simulink model "CSI_0313_SDC"  (R2019b)
settings: Solver=FixedStepDiscrete  StartTime=0.0  StopTime=Tstop  FixedStep=Tdelt  MaxStep=1e-4  RelTol=1e-3
values from neighbouring files (symbols this model uses):
  C = 12e-6    (= 1.2e-05)    [Inputparameter.m]
  Cdc = 4.76*10^-3    (= 0.00476)    [Inputparameter.m]
  Cemc = 1.5e-6    (= 1.5e-06)    [Inputparameter.m]
  enb = 0    [Run.m]
  fanalog = 7000    [Run.m]
  fTs = Update/18000    (= 0.000111111111111)    [Run.m]
  Ibase = 43*sqrt(2)    [Inputparameter.m]
  K120 = 0.0    (= 0)    [Run.m]
  K21 = 0.0    (= 0)    [Run.m]
  K5 = 0.0    (= 0)    [Run.m]
  K7 = 0.0    (= 0)    [Run.m]
  Kipll = 1.0    (= 1)    [Run.m]
  Klim = 1.03    [Run.m]
  Kpll = 20.0    (= 20)    [Run.m]
  Kpr = 0.9*Ibase/(Vbase)    [Run.m]
  Lgrid = 7.717e-4*10    (= 0.007717)    [Run.m]
  Lline = 60e-6    (= 6e-05)    [Inputparameter.m]
  Lpwm = 184.8e-6    (= 0.0001848)    [Inputparameter.m]
  mode = 1    [Run.m]
  Nsw = 18000/fbase    [Run.m]
  Qbpf = 1.0    (= 1)    [Run.m]
  Qpr = 1.0    (= 1)    [Run.m]
  Qs = 1    [Run.m]
  Rc = 10e-3    (= 0.01)    [Inputparameter.m]
  Remc = 1e-3    (= 0.001)    [Inputparameter.m]
  Rgrid = 2*pi*fbase*Lgrid/XR    [Run.m]
  Rline = 4.95e-3    (= 0.00495)    [Inputparameter.m]
  Rpre = 2.2    [Inputparameter.m]
  Rpwm = 6.2e-3    (= 0.0062)    [Inputparameter.m]
  Tdelt = (fTs)/(200*Update)    (= 2.77777777778e-07)    [Run.m]
  Tdt = 1.27e-6    (= 1.27e-06)    [Run.m]
  tstart = 0.2    [Run.m]
  Update = 2    [Run.m]
  Vbase = 400*sqrt(2/3)    [Inputparameter.m]
undefined symbols (not defined in the file or in its folder): sigbuilder_block
libraries: powerlib x54
(part 3 of 4)

== matlab function CSI_0313_SDC/AIP1/Subsystem7/Pos&Neg seq extract in subsystem /IIR_BPF_Re1 ==
  data: u input; fn input; fQ parameter; y output; fTs parameter; iMode parameter
function y =IIR_2rd(u, fn, fQ, fTs, iMode)
    % Second order transfer function used for LPF and BPF
    % y[n] = (fa1*x[n]+fa2*x[n-1]+fa3*x[n-2]-fb2*y[n-1]-fb3*y[n-2])/fb1
    % u:  error input
    % fn:  Natural frequency
    % fQ:   Quality factor
    % fTs:  Sampling time
    % iMode: Mode Selection
    % iMode=1 used as generalized 2nd-order LPF, LPF(s)=wn^2/(s^2+wn/Q*s+wn^2)
    % iMode=2 used as 2nd-order LPF in SOGI, SOGI_LPF(s)=(wn^2/Q)/(s^2+wn/Q*s+wn^2)
    % iMode=3 used as 2nd-order BPF in SOGI, SOGI_BPF(s)=(wn*s/Q)/(s^2+wn/Q*s+wn^2)
    
    persistent t;
    
    if isempty(t)
        t = zeros(2,3);
    end
    
    wn = 2*pi*fn;
    wc = wn/fQ;

    fT1 = wc*wn*fTs*fTs; 
    fT2 = 2*wc*fTs;
    fT3 = (wn*fTs)^2;
    
    fb1 = fT3+fT2+4;
    fb2 = 2*fT3-8;
    fb3 = fT3-fT2+4;
    
    if (iMode ==1)
        fa1 = fT3;
        fa2 = 2*fT3;
        fa3 = fT3;
    elseif (iMode ==2)
        fa1 = fT1;
        fa2 = 2*fT1;
        fa3 = fT1;
    else
        fa1 = fT2;
        fa2 = 0;
        fa3 = -fT2;
    end
%     if(Trigs > 0)
        t(1,1) = u;        
        t(2,1) = (fa1*t(1,1)+fa2*t(1,2)+fa3*t(1,3)-fb2*t(2,2)-fb3*t(2,3))/fb1;
    
        t(1,3) = t(1,2);
        t(1,2) = t(1,1);
        
        t(2,3) = t(2,2);
        t(2,2) = t(2,1);
%     else
%         t(1,1) = t(1,1);        
%         t(2,1) = t(2,1);
%     
%         t(1,3) = t(1,3);
%         t(1,2) = t(1,2);
%         
%         t(2,3) = t(2,3);
%         t(2,2) = t(2,2);
%     end
    
    y = t(2,1);    
end

== matlab function CSI_0313_SDC/AIP1/Subsystem7/Pos&Neg seq extract in subsystem /IIR_LPF_Im ==
  data: u input; fn input; fQ parameter; y output; fTs parameter; iMode parameter
function y =IIR_2rd(u, fn, fQ, fTs, iMode)
    % Second order transfer function used for LPF and BPF
    % y[n] = (fa1*x[n]+fa2*x[n-1]+fa3*x[n-2]-fb2*y[n-1]-fb3*y[n-2])/fb1
    % u:  error input
    % fn:  Natural frequency
    % fQ:   Quality factor
    % fTs:  Sampling time
    % iMode: Mode Selection
    % iMode=1 used as generalized 2nd-order LPF, LPF(s)=wn^2/(s^2+wn/Q*s+wn^2)
    % iMode=2 used as 2nd-order LPF in SOGI, SOGI_LPF(s)=(wn^2/Q)/(s^2+wn/Q*s+wn^2)
    % iMode=3 used as 2nd-order BPF in SOGI, SOGI_BPF(s)=(wn*s/Q)/(s^2+wn/Q*s+wn^2)
    
    persistent t;
    
    if isempty(t)
        t = zeros(2,3);
    end
    
    wn = 2*pi*fn;
    wc = wn/fQ;

    fT1 = wc*wn*fTs*fTs; 
    fT2 = 2*wc*fTs;
    fT3 = (wn*fTs)^2;
    
    fb1 = fT3+fT2+4;
    fb2 = 2*fT3-8;
    fb3 = fT3-fT2+4;
    
    if (iMode ==1)
        fa1 = fT3;
        fa2 = 2*fT3;
        fa3 = fT3;
    elseif (iMode ==2)
        fa1 = fT1;
        fa2 = 2*fT1;
        fa3 = fT1;
    else
        fa1 = fT2;
        fa2 = 0;
        fa3 = -fT2;
    end
        
%    if(Trigs > 0)
        t(1,1) = u;        
        t(2,1) = (fa1*t(1,1)+fa2*t(1,2)+fa3*t(1,3)-fb2*t(2,2)-fb3*t(2,3))/fb1;
    
        t(1,3) = t(1,2);
        t(1,2) = t(1,1);
        
        t(2,3) = t(2,2);
        t(2,2) = t(2,1);
%     else
%         t(1,1) = t(1,1);        
%         t(2,1) = t(2,1);
%     
%         t(1,3) = t(1,3);
%         t(1,2) = t(1,2);
%         
%         t(2,3) = t(2,3);
%         t(2,2) = t(2,2);
%     end
%     
    y = t(2,1);    
end

== matlab function CSI_0313_SDC/AIP1/Subsystem7/Current Limitation pu Standard/PI Ctrl ==
  data: err input; y output; fKI parameter; fMinLmt parameter; fTs parameter; fMaxLmt parameter; fKP parameter
function y = PICtrl(err, fKI, fMinLmt, fTs, fMaxLmt, fKP)
    % y[n] = y[n-1] + KP*(x[n]-x[n-1]) + (KP*KI*TS*0.5)*(x[n]+x[n-1])
    % err:  error input
    % fKP:   Proportional gain
    % fKI:   Integral Coefficient
    % fMinLmt: Minimum limitation
    % fMaxLmt: Maximum limitation
    % fTs:  Sampling time
    
    % t(1,2) stores x[n],x[n-1]; t(2,2) stores y[n],y[n-1]
    persistent t;      
    if isempty(t)           % Initialization
        t = zeros(2,2);
    end
    
%     if(Trig > 0)
        t(1,1) = err;
        t(2,1) = t(2,2) + fKP*(t(1,1)-t(1,2)) + fKP*fKI*0.5*(t(1,1)+t(1,2))*fTs;   
    
        if (t(2,1) < fMinLmt)
            t(2,1) = fMinLmt;
        elseif (t(2,1) > fMaxLmt)
            t(2,1) = fMaxLmt;
        end
    
        t(1,2) = t(1,1);
        t(2,2) = t(2,1);
%     else
%         t(1,1) = t(1,1);
%         t(2,1) = t(2,1);      
%         t(1,2) = t(1,2);
%         t(2,2) = t(2,2);
%     end
    y = t(2,1);
end

== matlab function CSI_0313_SDC/Programmal Grid/Programmal Grid  ==
  data: ua output; ub output; uc output; Tdelt parameter; K5 parameter; K7 parameter; K21 parameter; K120 parameter; t input
function [ua, ub, uc] = fcn(Tdelt,K5, K7, K21,K120,t)
persistent theta; 
 % Initialization
 if isempty(theta)           
    theta = pi/2;
 end 

f = 50;
Vm = 400*sqrt(2/3);
Tflt = 0.2;             %% fault duration time[s]
Vsag = 0.05 * Vm;        %% voltage level configuration during the fault
theta = theta + 2*pi*f*Tdelt;
if(theta >= 2*pi)
    theta = theta-2*pi;
end

Tinrpt = 12.21;
if (t < Tinrpt)
    Vol = Vm;
elseif (t>=Tinrpt && t<(Tinrpt+0.004))  %% the fault starts and ends in 4ms
    Vol = Vm-(t-Tinrpt)*(Vm - Vsag)/0.004;
elseif (t>=Tinrpt && t<(Tinrpt+0.004+Tflt)) %% the fault sustain Tflt[s]
    Vol = Vsag;
elseif (t>=(Tinrpt+0.004+Tflt) && t< (Tinrpt+0.008+Tflt))  %% the fault recoverys in 4ms
    Vol = Vsag+(t-(Tinrpt+0.004+Tflt))*(Vm - Vsag)/0.004;
else
    Vol = Vm;
end

ua = Vol*sin(theta)+K5*Vm*sin(5.0*theta)+K7*Vm*sin(7.0*theta)+K21*Vm*sin(21.0*theta)+K120*Vm*sin(120.0*theta);
ub = Vol*sin(theta-2*pi/3)+K5*Vm*sin(5.0*(theta-2*pi/3))+K7*Vm*sin(7.0*(theta-2*pi/3))+K120*Vm*sin(120.0*(theta-2*pi/3));
uc = Vol*sin(theta+2*pi/3)+K5*Vm*sin(5.0*(theta+2*pi/3))+K7*Vm*sin(7.0*(theta+2*pi/3))+K120*Vm*sin(120.0*(theta+2*pi/3));

end

== matlab function CSI_0313_SDC/AIP1/Subsystem7/Pos&Neg seq extract in subsystem /IIR_LPF_Re1 ==
  data: u input; fn input; fQ parameter; y output; fTs parameter; iMode parameter
function y =IIR_2rd(u, fn, fQ, fTs, iMode)
    % Second order transfer function used for LPF and BPF
    % y[n] = (fa1*x[n]+fa2*x[n-1]+fa3*x[n-2]-fb2*y[n-1]-fb3*y[n-2])/fb1
    % u:  error input
    % fn:  Natural frequency
    % fQ:   Quality factor
    % fTs:  Sampling time
    % iMode: Mode Selection
    % iMode=1 used as generalized 2nd-order LPF, LPF(s)=wn^2/(s^2+wn/Q*s+wn^2)
    % iMode=2 used as 2nd-order LPF in SOGI, SOGI_LPF(s)=(wn^2/Q)/(s^2+wn/Q*s+wn^2)
    % iMode=3 used as 2nd-order BPF in SOGI, SOGI_BPF(s)=(wn*s/Q)/(s^2+wn/Q*s+wn^2)
    
    persistent t;
    
    if isempty(t)
        t = zeros(2,3);
    end
    
    wn = 2*pi*fn;
    wc = wn/fQ;

    fT1 = wc*wn*fTs*fTs; 
    fT2 = 2*wc*fTs;
    fT3 = (wn*fTs)^2;
    
    fb1 = fT3+fT2+4;
    fb2 = 2*fT3-8;
    fb3 = fT3-fT2+4;
    
    if (iMode ==1)
        fa1 = fT3;
        fa2 = 2*fT3;
        fa3 = fT3;
    elseif (iMode ==2)
        fa1 = fT1;
        fa2 = 2*fT1;
        fa3 = fT1;
    else
        fa1 = fT2;
        fa2 = 0;
        fa3 = -fT2;
    end
        
%    if(Trigs > 0)
        t(1,1) = u;        
        t(2,1) = (fa1*t(1,1)+fa2*t(1,2)+fa3*t(1,3)-fb2*t(2,2)-fb3*t(2,3))/fb1;
    
        t(1,3) = t(1,2);
        t(1,2) = t(1,1);
        
        t(2,3) = t(2,2);
        t(2,2) = t(2,1);
%     else
%         t(1,1) = t(1,1);        
%         t(2,1) = t(2,1);
%     
%         t(1,3) = t(1,3);
%         t(1,2) = t(1,2);
%         
%         t(2,3) = t(2,3);
%         t(2,2) = t(2,2);
%     end
    
    y = t(2,1);    
end

== matlab function CSI_0313_SDC/AIP1/Subsystem7/Pos&Neg seq extract in subsystem 1/IIR_BPF_Im ==
  data: u input; fn input; fQ parameter; y output; fTs parameter; iMode parameter
function y =IIR_2rd(u, fn, fQ, fTs, iMode)
    % Second order transfer function used for LPF and BPF
    % y[n] = (fa1*x[n]+fa2*x[n-1]+fa3*x[n-2]-fb2*y[n-1]-fb3*y[n-2])/fb1
    % u:  error input
    % fn:  Natural frequency
    % fQ:   Quality factor
    % fTs:  Sampling time
    % iMode: Mode Selection
    % iMode=1 used as generalized 2nd-order LPF, LPF(s)=wn^2/(s^2+wn/Q*s+wn^2)
    % iMode=2 used as 2nd-order LPF in SOGI, SOGI_LPF(s)=(wn^2/Q)/(s^2+wn/Q*s+wn^2)
    % iMode=3 used as 2nd-order BPF in SOGI, SOGI_BPF(s)=(wn*s/Q)/(s^2+wn/Q*s+wn^2)
    
    persistent t;
    
    if isempty(t)
        t = zeros(2,3);
    end
    
    wn = 2*pi*fn;
    wc = wn/fQ;

    fT1 = wc*wn*fTs*fTs; 
    fT2 = 2*wc*fTs;
    fT3 = (wn*fTs)^2;
    
    fb1 = fT3+fT2+4;
    fb2 = 2*fT3-8;
    fb3 = fT3-fT2+4;
    
    if (iMode ==1)
        fa1 = fT3;
        fa2 = 2*fT3;
        fa3 = fT3;
    elseif (iMode ==2)
        fa1 = fT1;
        fa2 = 2*fT1;
        fa3 = fT1;
    else
        fa1 = fT2;
        fa2 = 0;
        fa3 = -fT2;
    end
        
%     if(Trigs > 0)
        t(1,1) = u;        
        t(2,1) = (fa1*t(1,1)+fa2*t(1,2)+fa3*t(1,3)-fb2*t(2,2)-fb3*t(2,3))/fb1;
    
        t(1,3) = t(1,2);
        t(1,2) = t(1,1);
        
        t(2,3) = t(2,2);
        t(2,2) = t(2,1);
%     else
%         t(1,1) = t(1,1);        
%         t(2,1) = t(2,1);
%     
%         t(1,3) = t(1,3);
%         t(1,2) = t(1,2);
%         
%         t(2,3) = t(2,3);
%         t(2,2) = t(2,2);
%     end
    
    y = t(2,1);    
end

== matlab function CSI_0313_SDC/AIP1/Subsystem7/Current Limitation pu Standard/PI Ctrl2 ==
  data: err input; y output; fKI parameter; fMinLmt parameter; fTs parameter; fMaxLmt parameter; fKP parameter
function y = PICtrl(err, fKI, fMinLmt, fTs, fMaxLmt, fKP)
    % y[n] = y[n-1] + KP*(x[n]-x[n-1]) + (KP*KI*TS*0.5)*(x[n]+x[n-1])
    % err:  error input
    % fKP:   Proportional gain
    % fKI:   Integral Coefficient
    % fMinLmt: Minimum limitation
    % fMaxLmt: Maximum limitation
    % fTs:  Sampling time
    
    % t(1,2) stores x[n],x[n-1]; t(2,2) stores y[n],y[n-1]
    persistent t;      
    if isempty(t)           % Initialization
        t = zeros(2,2);
    end
    
%     if(Trig > 0)
        t(1,1) = err;
        t(2,1) = t(2,2) + fKP*(t(1,1)-t(1,2)) + fKP*fKI*0.5*(t(1,1)+t(1,2))*fTs;   
    
        if (t(2,1) < fMinLmt)
            t(2,1) = fMinLmt;
        elseif (t(2,1) > fMaxLmt)
            t(2,1) = fMaxLmt;
        end
    
        t(1,2) = t(1,1);
        t(2,2) = t(2,1);
%     else
%         t(1,1) = t(1,1);
%         t(2,1) = t(2,1);      
%         t(1,2) = t(1,2);
%         t(2,2) = t(2,2);
%     end
    y = t(2,1);
end

== matlab function CSI_0313_SDC/AIP1/Subsystem7/Pos&Neg seq extract in subsystem 1/IIR_BPF_Re1 ==
  data: u input; fn input; fQ parameter; y output; fTs parameter; iMode parameter
function y =IIR_2rd(u, fn, fQ, fTs, iMode)
    % Second order transfer function used for LPF and BPF
    % y[n] = (fa1*x[n]+fa2*x[n-1]+fa3*x[n-2]-fb2*y[n-1]-fb3*y[n-2])/fb1
    % u:  error input
    % fn:  Natural frequency
    % fQ:   Quality factor
    % fTs:  Sampling time
    % iMode: Mode Selection
    % iMode=1 used as generalized 2nd-order LPF, LPF(s)=wn^2/(s^2+wn/Q*s+wn^2)
    % iMode=2 used as 2nd-order LPF in SOGI, SOGI_LPF(s)=(wn^2/Q)/(s^2+wn/Q*s+wn^2)
    % iMode=3 used as 2nd-order BPF in SOGI, SOGI_BPF(s)=(wn*s/Q)/(s^2+wn/Q*s+wn^2)
    
    persistent t;
    
    if isempty(t)
        t = zeros(2,3);
    end
    
    wn = 2*pi*fn;
    wc = wn/fQ;

    fT1 = wc*wn*fTs*fTs; 
    fT2 = 2*wc*fTs;
    fT3 = (wn*fTs)^2;
    
    fb1 = fT3+fT2+4;
    fb2 = 2*fT3-8;
    fb3 = fT3-fT2+4;
    
    if (iMode ==1)
        fa1 = fT3;
        fa2 = 2*fT3;
        fa3 = fT3;
    elseif (iMode ==2)
        fa1 = fT1;
        fa2 = 2*fT1;
        fa3 = fT1;
    else
        fa1 = fT2;
        fa2 = 0;
        fa3 = -fT2;
    end
%     if(Trigs > 0)
        t(1,1) = u;        
        t(2,1) = (fa1*t(1,1)+fa2*t(1,2)+fa3*t(1,3)-fb2*t(2,2)-fb3*t(2,3))/fb1;
    
        t(1,3) = t(1,2);
        t(1,2) = t(1,1);
        
        t(2,3) = t(2,2);
        t(2,2) = t(2,1);
%     else
%         t(1,1) = t(1,1);        
%         t(2,1) = t(2,1);
%     
%         t(1,3) = t(1,3);
%         t(1,2) = t(1,2);
%         
%         t(2,3) = t(2,3);
%         t(2,2) = t(2,2);
%     end
    
    y = t(2,1);    
end

== matlab function CSI_0313_SDC/AIP1/Subsystem7/Pos&Neg seq extract in subsystem 1/IIR_LPF_Im ==
  data: u input; fn input; fQ parameter; y output; fTs parameter; iMode parameter
function y =IIR_2rd(u, fn, fQ, fTs, iMode)
    % Second order transfer function used for LPF and BPF
    % y[n] = (fa1*x[n]+fa2*x[n-1]+fa3*x[n-2]-fb2*y[n-1]-fb3*y[n-2])/fb1
    % u:  error input
    % fn:  Natural frequency
    % fQ:   Quality factor
    % fTs:  Sampling time
    % iMode: Mode Selection
    % iMode=1 used as generalized 2nd-order LPF, LPF(s)=wn^2/(s^2+wn/Q*s+wn^2)
    % iMode=2 used as 2nd-order LPF in SOGI, SOGI_LPF(s)=(wn^2/Q)/(s^2+wn/Q*s+wn^2)
    % iMode=3 used as 2nd-order BPF in SOGI, SOGI_BPF(s)=(wn*s/Q)/(s^2+wn/Q*s+wn^2)
    
    persistent t;
    
    if isempty(t)
        t = zeros(2,3);
    end
    
    wn = 2*pi*fn;
    wc = wn/fQ;

    fT1 = wc*wn*fTs*fTs; 
    fT2 = 2*wc*fTs;
    fT3 = (wn*fTs)^2;
    
    fb1 = fT3+fT2+4;
    fb2 = 2*fT3-8;
    fb3 = fT3-fT2+4;
    
    if (iMode ==1)
        fa1 = fT3;
        fa2 = 2*fT3;
        fa3 = fT3;
    elseif (iMode ==2)
        fa1 = fT1;
        fa2 = 2*fT1;
        fa3 = fT1;
    else
        fa1 = fT2;
        fa2 = 0;
        fa3 = -fT2;
    end
        
%    if(Trigs > 0)
        t(1,1) = u;        
        t(2,1) = (fa1*t(1,1)+fa2*t(1,2)+fa3*t(1,3)-fb2*t(2,2)-fb3*t(2,3))/fb1;
    
        t(1,3) = t(1,2);
        t(1,2) = t(1,1);
        
        t(2,3) = t(2,2);
        t(2,2) = t(2,1);
%     else
%         t(1,1) = t(1,1);        
%         t(2,1) = t(2,1);
%     
%         t(1,3) = t(1,3);
%         t(1,2) = t(1,2);
%         
%         t(2,3) = t(2,3);
%         t(2,2) = t(2,2);
%     end
%     
    y = t(2,1);    
end

== matlab function CSI_0313_SDC/AIP1/VLine_To_VPh ==
  data: VLine input; VPh output
function VPh = VLine_To_VPh(VLine)
    % Assume Van+Vbn+Vcn=0
    % VLine(1)=Vab; VLine(2)=Vbc; VLine(3)=Vca 
    % VPh(1)=Van; VPh(2)=Vbn; VPh(3)=Vcn;
    VPh = [0;0;0];
    VPh(1) = (VLine(1)-VLine(3))/3;
    VPh(2) = (VLine(2)-VLine(1))/3;
    VPh(3) = (VLine(3)-VLine(2))/3;
end

== matlab function CSI_0313_SDC/AIP1/Subsystem7/Pos&Neg seq extract in subsystem 1/IIR_LPF_Re1 ==
  data: u input; fn input; fQ parameter; y output; fTs parameter; iMode parameter
function y =IIR_2rd(u, fn, fQ, fTs, iMode)
    % Second order transfer function used for LPF and BPF
    % y[n] = (fa1*x[n]+fa2*x[n-1]+fa3*x[n-2]-fb2*y[n-1]-fb3*y[n-2])/fb1
    % u:  error input
    % fn:  Natural frequency
    % fQ:   Quality factor
    % fTs:  Sampling time
    % iMode: Mode Selection
    % iMode=1 used as generalized 2nd-order LPF, LPF(s)=wn^2/(s^2+wn/Q*s+wn^2)
    % iMode=2 used as 2nd-order LPF in SOGI, SOGI_LPF(s)=(wn^2/Q)/(s^2+wn/Q*s+wn^2)
    % iMode=3 used as 2nd-order BPF in SOGI, SOGI_BPF(s)=(wn*s/Q)/(s^2+wn/Q*s+wn^2)
    
    persistent t;
    
    if isempty(t)
        t = zeros(2,3);
    end
    
    wn = 2*pi*fn;
    wc = wn/fQ;

    fT1 = wc*wn*fTs*fTs; 
    fT2 = 2*wc*fTs;
    fT3 = (wn*fTs)^2;
    
    fb1 = fT3+fT2+4;
    fb2 = 2*fT3-8;
    fb3 = fT3-fT2+4;
    
    if (iMode ==1)
        fa1 = fT3;
        fa2 = 2*fT3;
        fa3 = fT3;
    elseif (iMode ==2)
        fa1 = fT1;
        fa2 = 2*fT1;
        fa3 = fT1;
    else
        fa1 = fT2;
        fa2 = 0;
        fa3 = -fT2;
    end
        
%    if(Trigs > 0)
        t(1,1) = u;        
        t(2,1) = (fa1*t(1,1)+fa2*t(1,2)+fa3*t(1,3)-fb2*t(2,2)-fb3*t(2,3))/fb1;
    
        t(1,3) = t(1,2);
        t(1,2) = t(1,1);
        
        t(2,3) = t(2,2);
        t(2,2) = t(2,1);
%     else
%         t(1,1) = t(1,1);        
%         t(2,1) = t(2,1);
%     
%         t(1,3) = t(1,3);
%         t(1,2) = t(1,2);
%         
%         t(2,3) = t(2,3);
%         t(2,2) = t(2,2);
%     end
    
    y = t(2,1);    
end

== matlab function CSI_0313_SDC/AIP1/Moving average ==
  data: yout output; uin input; trig input; iNumAvg parameter; iNumDly parameter; ubase parameter
function yout=sample(uin,trig,iNumAvg,iNumDly,ubase)

persistent uary cnt sum yavg;

iNumIn = length(uin);
iNumDly = iNumDly+1;
if isempty(cnt)  
    cnt = 0;
    uary = zeros(iNumIn,iNumAvg);
    sum = zeros(iNumIn,1);
    yavg = zeros(iNumIn,iNumDly);   
end

if(trig >0) 
    for i=1:1:iNumIn
        for j=iNumDly:-1:2
            yavg(i,j)= yavg(i,j-1);
        end
    end
    cnt = cnt +1;
    for i=1:1:iNumIn
         uary(i,cnt) = uin(i)/ubase;            
        for j=1:1:iNumAvg
        sum(i) = sum(i)+uary(i,j);
        end
    end
       for i=1:1:iNumIn
            yavg(i,1)=sum(i)/iNumAvg;
       end
        
        for i=1:1:iNumIn
            sum(i)=0;
        end
        if(cnt >= iNumAvg)
            cnt = 0;
        end
end
    yout = yavg(:,iNumDly);
end

== matlab function CSI_0313_SDC/AIP1/Subsystem7/Current Limitation pu Standard/PI Ctrl3 ==
  data: err input; y output; fKI parameter; fMinLmt parameter; fTs parameter; fMaxLmt parameter; fKP parameter
function y = PICtrl(err, fKI, fMinLmt, fTs, fMaxLmt, fKP)
    % y[n] = y[n-1] + KP*(x[n]-x[n-1]) + (KP*KI*TS*0.5)*(x[n]+x[n-1])
    % err:  error input
    % fKP:   Proportional gain
    % fKI:   Integral Coefficient
    % fMinLmt: Minimum limitation
    % fMaxLmt: Maximum limitation
    % fTs:  Sampling time
    
    % t(1,2) stores x[n],x[n-1]; t(2,2) stores y[n],y[n-1]
    persistent t;      
    if isempty(t)           % Initialization
        t = zeros(2,2);
    end
    
%     if(Trig > 0)
        t(1,1) = err;
        t(2,1) = t(2,2) + fKP*(t(1,1)-t(1,2)) + fKP*fKI*0.5*(t(1,1)+t(1,2))*fTs;   
    
        if (t(2,1) < fMinLmt)
            t(2,1) = fMinLmt;
        elseif (t(2,1) > fMaxLmt)
            t(2,1) = fMaxLmt;
        end
    
        t(1,2) = t(1,1);
        t(2,2) = t(2,1);
%     else
%         t(1,1) = t(1,1);
%         t(2,1) = t(2,1);      
%         t(1,2) = t(1,2);
%         t(2,2) = t(2,2);
%     end
    y = t(2,1);
end

== matlab function CSI_0313_SDC/AIP1/Moving average1 ==
  data: yout output; uin input; trig input; iNumAvg parameter; iNumDly parameter; ubase parameter
function yout=sample(uin,trig,iNumAvg,iNumDly,ubase)

persistent uary cnt sum yavg;

iNumIn = length(uin);
iNumDly = iNumDly+1;
if isempty(cnt)  
    cnt = 0;
    uary = zeros(iNumIn,iNumAvg);
    sum = zeros(iNumIn,1);
    yavg = zeros(iNumIn,iNumDly);   
end

if(trig >0) 
    for i=1:1:iNumIn
        for j=iNumDly:-1:2
            yavg(i,j)= yavg(i,j-1);
        end
    end
    cnt = cnt +1;
    for i=1:1:iNumIn
         uary(i,cnt) = uin(i)/ubase;            
        for j=1:1:iNumAvg
        sum(i) = sum(i)+uary(i,j);
        end
    end
       for i=1:1:iNumIn
            yavg(i,1)=sum(i)/iNumAvg;
       end
        
        for i=1:1:iNumIn
            sum(i)=0;
        end
        if(cnt >= iNumAvg)
            cnt = 0;
        end
end
    yout = yavg(:,iNumDly);
end

== matlab function CSI_0313_SDC/AIP1/Sample//Moving window1 ==
  data: yout output; uin input; trig input; iNumAvg parameter; iNumDly parameter; ubase parameter
function yout=sample(uin,trig,iNumAvg,iNumDly,ubase)

persistent uary cnt sum yavg;

iNumIn = length(uin);
iNumDly = iNumDly+1;
if isempty(cnt)  
    cnt = 0;
    uary = zeros(iNumIn,iNumAvg);
    sum = zeros(iNumIn,1);
    yavg = zeros(iNumIn,iNumDly);    
end

if(trig >0) 
    for i=1:1:iNumIn
        for j=iNumDly:-1:2
            yavg(i,j)= yavg(i,j-1);
        end
    end
    cnt = cnt +1;
    for i=1:1:iNumIn
        uary(i,cnt) = uin(i)/ubase;
        sum(i) = sum(i)+uary(i,cnt);
    end
    if(cnt == iNumAvg)
        cnt = 0;
        for i=1:1:iNumIn
            yavg(i,1)=sum(i)/iNumAvg;
        end
        for i=1:1:iNumIn
            sum(i)=0;
        end
    end        
end
    yout = yavg(:,iNumDly);
end

== matlab function CSI_0313_SDC/AIP1/Subsystem7/Current Limitation pu Standard/RMS ==
  data: u input; y output; iNumAry parameter
function y = RMS(u, iNumAry)
% Calculate the RMS value of input with the window points of iNumAry
    persistent sum cnt uary;
    % Initialization
    if isempty(sum)
            sum = 0;
            cnt = 1;
            uary = zeros(iNumAry,1);
    end
    
    usqr = u*u;                 % Square calculation
    sum = sum+usqr-uary(cnt);   % Sum of the square
    uary(cnt) = usqr;           % Update the latest square
    
    if(sum<=0)
        sum=0;
    end
    y = sqrt(sum/iNumAry);      % RMS value
    % Update the counter of square array
    if(cnt < iNumAry)
        cnt = cnt + 1;
    else
        cnt = 1;
    end
end

== matlab function CSI_0313_SDC/AIP1/Subsystem7/Current Limitation pu Standard/RMS1 ==
  data: u input; y output; iNumAry parameter
function y = RMS(u, iNumAry)
% Calculate the RMS value of input with the window points of iNumAry
    persistent sum cnt uary;
    % Initialization
    if isempty(sum)
            sum = 0;
            cnt = 1;
            uary = zeros(iNumAry,1);
    end
    
    usqr = u*u;                 % Square calculation
    sum = sum+usqr-uary(cnt);   % Sum of the square
    uary(cnt) = usqr;           % Update the latest square
    
    if(sum<=0)
        sum=0;
    end
    y = sqrt(sum/iNumAry);      % RMS value
    % Update the counter of square array
    if(cnt < iNumAry)
        cnt = cnt + 1;
    else
        cnt = 1;
    end
end

== matlab function CSI_0313_SDC/AIP1/Subsystem7/Current Limitation pu Standard/RMS2 ==
  data: u input; y output; iNumAry parameter
function y = RMS(u, iNumAry)
% Calculate the RMS value of input with the window points of iNumAry
    persistent sum cnt uary;
    % Initialization
    if isempty(sum)
            sum = 0;
            cnt = 1;
            uary = zeros(iNumAry,1);
    end
    
    usqr = u*u;                 % Square calculation
    sum = sum+usqr-uary(cnt);   % Sum of the square
    uary(cnt) = usqr;           % Update the latest square
    
    if(sum<=0)
        sum=0;
    end
    y = sqrt(sum/iNumAry);      % RMS value
    % Update the counter of square array
    if(cnt < iNumAry)
        cnt = cnt + 1;
    else
        cnt = 1;
    end
end

== matlab function CSI_0313_SDC/AIP1/Subsystem7/ABC_To_RIZ2 ==
  data: ABC input; RIZ output
function RIZ = ABC_To_RIZ(ABC)
    % Clarke Transfer from ABC axis to Re-Im axis
    RIZ = [0;0;0];
    RIZ(1) = (2*ABC(1)-ABC(2)-ABC(3))/3;
    RIZ(2) = sqrt(3)*(ABC(2)-ABC(3))/3;
    RIZ(3) = (ABC(1)+ABC(2)+ABC(3))/3;
end

== matlab function CSI_0313_SDC/AIP1/Subsystem7/Current Limitation pu Standard/RMS3 ==
  data: u input; y output; iNumAry parameter
function y = RMS(u, iNumAry)
% Calculate the RMS value of input with the window points of iNumAry
    persistent sum cnt uary;
    % Initialization
    if isempty(sum)
            sum = 0;
            cnt = 1;
            uary = zeros(iNumAry,1);
    end
    
    usqr = u*u;                 % Square calculation
    sum = sum+usqr-uary(cnt);   % Sum of the square
    uary(cnt) = usqr;           % Update the latest square
    
    if(sum<=0)
        sum=0;
    end
    y = sqrt(sum/iNumAry);      % RMS value
    % Update the counter of square array
    if(cnt < iNumAry)
        cnt = cnt + 1;
    else
        cnt = 1;
    end
end

== matlab function CSI_0313_SDC/AIP1/Subsystem7/PLL/RIZ_To_DQ0 ==
  data: RIZ input; DQ0 output; wt input; iAxis parameter
function DQ0 = RIZ_To_DQ0(RIZ,wt,iAxis)
    % Park Transfer from Re-Im axis to DQ0 axis
    DQ0 = [0;0;0];
    if (iAxis == 1)
        DQ0(1) = RIZ(1)*cos(wt)+RIZ(2)*sin(wt);
        DQ0(2) = -RIZ(1)*sin(wt)+RIZ(2)*cos(wt);
    else
        DQ0(1) = RIZ(1)*sin(wt)-RIZ(2)*cos(wt);
        DQ0(2) = RIZ(1)*cos(wt)+RIZ(2)*sin(wt);
    end
end

== matlab function CSI_0313_SDC/AIP1/Subsystem7/Pos&Neg seq extract in subsystem 2/IIR_BPF_Im ==
  data: u input; fn input; fQ parameter; y output; fTs parameter; iMode parameter
function y =IIR_2rd(u, fn, fQ, fTs, iMode)
    % Second order transfer function used for LPF and BPF
    % y[n] = (fa1*x[n]+fa2*x[n-1]+fa3*x[n-2]-fb2*y[n-1]-fb3*y[n-2])/fb1
    % u:  error input
    % fn:  Natural frequency
    % fQ:   Quality factor
    % fTs:  Sampling time
    % iMode: Mode Selection
    % iMode=1 used as generalized 2nd-order LPF, LPF(s)=wn^2/(s^2+wn/Q*s+wn^2)
    % iMode=2 used as 2nd-order LPF in SOGI, SOGI_LPF(s)=(wn^2/Q)/(s^2+wn/Q*s+wn^2)
    % iMode=3 used as 2nd-order BPF in SOGI, SOGI_BPF(s)=(wn*s/Q)/(s^2+wn/Q*s+wn^2)
    
    persistent t;
    
    if isempty(t)
        t = zeros(2,3);
    end
    
    wn = 2*pi*fn;
    wc = wn/fQ;

    fT1 = wc*wn*fTs*fTs; 
    fT2 = 2*wc*fTs;
    fT3 = (wn*fTs)^2;
    
    fb1 = fT3+fT2+4;
    fb2 = 2*fT3-8;
    fb3 = fT3-fT2+4;
    
    if (iMode ==1)
        fa1 = fT3;
        fa2 = 2*fT3;
        fa3 = fT3;
    elseif (iMode ==2)
        fa1 = fT1;
        fa2 = 2*fT1;
        fa3 = fT1;
    else
        fa1 = fT2;
        fa2 = 0;
        fa3 = -fT2;
    end
        
%     if(Trigs > 0)
        t(1,1) = u;        
        t(2,1) = (fa1*t(1,1)+fa2*t(1,2)+fa3*t(1,3)-fb2*t(2,2)-fb3*t(2,3))/fb1;
    
        t(1,3) = t(1,2);
        t(1,2) = t(1,1);
        
        t(2,3) = t(2,2);
        t(2,2) = t(2,1);
%     else
%         t(1,1) = t(1,1);        
%         t(2,1) = t(2,1);
%     
%         t(1,3) = t(1,3);
%         t(1,2) = t(1,2);
%         
%         t(2,3) = t(2,3);
%         t(2,2) = t(2,2);
%     end
    
    y = t(2,1);    
end

== matlab function CSI_0313_SDC/AIP1/Subsystem7/Pos&Neg seq extract in subsystem 2/IIR_BPF_Re1 ==
  data: u input; fn input; fQ parameter; y output; fTs parameter; iMode parameter
function y =IIR_2rd(u, fn, fQ, fTs, iMode)
    % Second order transfer function used for LPF and BPF
    % y[n] = (fa1*x[n]+fa2*x[n-1]+fa3*x[n-2]-fb2*y[n-1]-fb3*y[n-2])/fb1
    % u:  error input
    % fn:  Natural frequency
    % fQ:   Quality factor
    % fTs:  Sampling time
    % iMode: Mode Selection
    % iMode=1 used as generalized 2nd-order LPF, LPF(s)=wn^2/(s^2+wn/Q*s+wn^2)
    % iMode=2 used as 2nd-order LPF in SOGI, SOGI_LPF(s)=(wn^2/Q)/(s^2+wn/Q*s+wn^2)
    % iMode=3 used as 2nd-order BPF in SOGI, SOGI_BPF(s)=(wn*s/Q)/(s^2+wn/Q*s+wn^2)
    
    persistent t;
    
    if isempty(t)
        t = zeros(2,3);
    end
    
    wn = 2*pi*fn;
    wc = wn/fQ;

    fT1 = wc*wn*fTs*fTs; 
    fT2 = 2*wc*fTs;
    fT3 = (wn*fTs)^2;
    
    fb1 = fT3+fT2+4;
    fb2 = 2*fT3-8;
    fb3 = fT3-fT2+4;
    
    if (iMode ==1)
        fa1 = fT3;
        fa2 = 2*fT3;
        fa3 = fT3;
    elseif (iMode ==2)
        fa1 = fT1;
        fa2 = 2*fT1;
        fa3 = fT1;
    else
        fa1 = fT2;
        fa2 = 0;
        fa3 = -fT2;
    end
%     if(Trigs > 0)
        t(1,1) = u;        
        t(2,1) = (fa1*t(1,1)+fa2*t(1,2)+fa3*t(1,3)-fb2*t(2,2)-fb3*t(2,3))/fb1;
    
        t(1,3) = t(1,2);
        t(1,2) = t(1,1);
        
        t(2,3) = t(2,2);
        t(2,2) = t(2,1);
%     else
%         t(1,1) = t(1,1);        
%         t(2,1) = t(2,1);
%     
%         t(1,3) = t(1,3);
%         t(1,2) = t(1,2);
%         
%         t(2,3) = t(2,3);
%         t(2,2) = t(2,2);
%     end
    
    y = t(2,1);    
end

== matlab function CSI_0313_SDC/AIP1/Subsystem7/Pos&Neg seq extract in subsystem 2/IIR_LPF_Im ==
  data: u input; fn input; fQ parameter; y output; fTs parameter; iMode parameter
function y =IIR_2rd(u, fn, fQ, fTs, iMode)
    % Second order transfer function used for LPF and BPF
    % y[n] = (fa1*x[n]+fa2*x[n-1]+fa3*x[n-2]-fb2*y[n-1]-fb3*y[n-2])/fb1
    % u:  error input
    % fn:  Natural frequency
    % fQ:   Quality factor
    % fTs:  Sampling time
    % iMode: Mode Selection
    % iMode=1 used as generalized 2nd-order LPF, LPF(s)=wn^2/(s^2+wn/Q*s+wn^2)
    % iMode=2 used as 2nd-order LPF in SOGI, SOGI_LPF(s)=(wn^2/Q)/(s^2+wn/Q*s+wn^2)
    % iMode=3 used as 2nd-order BPF in SOGI, SOGI_BPF(s)=(wn*s/Q)/(s^2+wn/Q*s+wn^2)
    
    persistent t;
    
    if isempty(t)
        t = zeros(2,3);
    end
    
    wn = 2*pi*fn;
    wc = wn/fQ;

    fT1 = wc*wn*fTs*fTs; 
    fT2 = 2*wc*fTs;
    fT3 = (wn*fTs)^2;
    
    fb1 = fT3+fT2+4;
    fb2 = 2*fT3-8;
    fb3 = fT3-fT2+4;
    
    if (iMode ==1)
        fa1 = fT3;
        fa2 = 2*fT3;
        fa3 = fT3;
    elseif (iMode ==2)
        fa1 = fT1;
        fa2 = 2*fT1;
        fa3 = fT1;
    else
        fa1 = fT2;
        fa2 = 0;
        fa3 = -fT2;
    end
        
%    if(Trigs > 0)
        t(1,1) = u;        
        t(2,1) = (fa1*t(1,1)+fa2*t(1,2)+fa3*t(1,3)-fb2*t(2,2)-fb3*t(2,3))/fb1;
    
        t(1,3) = t(1,2);
        t(1,2) = t(1,1);
        
        t(2,3) = t(2,2);
        t(2,2) = t(2,1);
%     else
%         t(1,1) = t(1,1);        
%         t(2,1) = t(2,1);
%     
%         t(1,3) = t(1,3);
%         t(1,2) = t(1,2);
%         
%         t(2,3) = t(2,3);
%         t(2,2) = t(2,2);
%     end
%     
    y = t(2,1);    
end

== matlab function CSI_0313_SDC/AIP1/Subsystem7/PR CSI Loop/PR Ctrl1 ==
  data: err input; y output; ffc input; fP parameter; fQ parameter; fTs parameter
function y = PRCtrl(err, ffc, fP, fQ, fTs)
    % PR regulation with variant frequency input
    % y[n] = (fa1*x[n]+fa2*x[n-1]+fa3*x[n-2]-fb2*y[n-1]-fb3*y[n-2])/fb1
    % err:  error input
    % ffc:  Natural frequency
    % fP:   Proportional gain
    % fQ:   Quality factor
    % fTs:  Sampling time
    
    % t(1,3) stores x[n],x[n-1],x[n-2]; t(2,3) stores y[n],y[n-1],y[n-2]
    persistent t;      
    if isempty(t)           % Initialization
        t = zeros(2,3);
    end

    fwc = 2*pi*ffc;
    fw0 = fwc/fQ;
    
    fT1 = 2*fw0*fTs;            
    fT2 = (fwc*fTs)^2;  

    fa1 = (4+fT1+fT2)*fP;
    fa2 = (2*fT2-8)*fP;
    fa3 = (4-fT1+fT2)*fP;
    fb1 = 4+fT2;
    fb2 = 2*fT2-8;
    fb3 = 4+fT2;
%     if(Trig > 0)
        t(1,1) = err;
        t(2,1) = (fa1*t(1,1)+fa2*t(1,2)+fa3*t(1,3)-fb2*t(2,2)-fb3*t(2,3))/fb1;     
        
        t(1,3) = t(1,2);
        t(1,2) = t(1,1);
 
        t(2,3) = t(2,2);
        t(2,2) = t(2,1);
%     else
%         t(1,1) = t(1,1);
%         t(2,1) = t(2,1);     
%         
%         t(1,3) = t(1,3);
%         t(1,2) = t(1,2);
%  
%         t(2,3) = t(2,3);
%         t(2,2) = t(2,2);
%         
%     end
    y = t(2,1);
end

== matlab function CSI_0313_SDC/AIP1/Subsystem7/PR CSI Loop/PR Ctrl2 ==
  data: err input; y output; ffc input; fP parameter; fQ parameter; fTs parameter
function y = PRCtrl(err, ffc, fP, fQ, fTs)
    % PR regulation with variant frequency input
    % y[n] = (fa1*x[n]+fa2*x[n-1]+fa3*x[n-2]-fb2*y[n-1]-fb3*y[n-2])/fb1
    % err:  error input
    % ffc:  Natural frequency
    % fP:   Proportional gain
    % fQ:   Quality factor
    % fTs:  Sampling time
    
    % t(1,3) stores x[n],x[n-1],x[n-2]; t(2,3) stores y[n],y[n-1],y[n-2]
    persistent t;      
    if isempty(t)           % Initialization
        t = zeros(2,3);
    end

    fwc = 2*pi*ffc;
    fw0 = fwc/fQ;
    
    fT1 = 2*fw0*fTs;            
    fT2 = (fwc*fTs)^2;  

    fa1 = (4+fT1+fT2)*fP;
    fa2 = (2*fT2-8)*fP;
    fa3 = (4-fT1+fT2)*fP;
    fb1 = 4+fT2;
    fb2 = 2*fT2-8;
    fb3 = 4+fT2;
    
%     if(Trig > 0)
        t(1,1) = err;
        t(2,1) = (fa1*t(1,1)+fa2*t(1,2)+fa3*t(1,3)-fb2*t(2,2)-fb3*t(2,3))/fb1;     
        
        t(1,3) = t(1,2);
        t(1,2) = t(1,1);
 
        t(2,3) = t(2,2);
        t(2,2) = t(2,1);
%     else
%         t(1,1) = t(1,1);
%         t(2,1) = t(2,1);     
%         
%         t(1,3) = t(1,3);
%         t(1,2) = t(1,2);
%  
%         t(2,3) = t(2,3);
%         t(2,2) = t(2,2);        
%     end
    
    y = t(2,1);
end

== matlab function CSI_0313_SDC/AIP1/Subsystem7/PR CSI Loop/RIZ_To_ABC ==
  data: RIZ input; ABC output
function ABC = RIZ_To_ABC(RIZ)
    % Inverse Clarke Transfer from Re-Im axis to ABC axis
    ABC = [0;0;0];
    ABC(1) = RIZ(1)+RIZ(3);
    ABC(2) = -(RIZ(1)-sqrt(3)*RIZ(2))/2+RIZ(3);
    ABC(3) = -(RIZ(1)+sqrt(3)*RIZ(2))/2+RIZ(3);
end

== matlab function CSI_0313_SDC/AIP1/Subsystem7/Pos&Neg seq extract in subsystem 2/IIR_LPF_Re1 ==
  data: u input; fn input; fQ parameter; y output; fTs parameter; iMode parameter
function y =IIR_2rd(u, fn, fQ, fTs, iMode)
    % Second order transfer function used for LPF and BPF
    % y[n] = (fa1*x[n]+fa2*x[n-1]+fa3*x[n-2]-fb2*y[n-1]-fb3*y[n-2])/fb1
    % u:  error input
    % fn:  Natural frequency
    % fQ:   Quality factor
    % fTs:  Sampling time
    % iMode: Mode Selection
    % iMode=1 used as generalized 2nd-order LPF, LPF(s)=wn^2/(s^2+wn/Q*s+wn^2)
    % iMode=2 used as 2nd-order LPF in SOGI, SOGI_LPF(s)=(wn^2/Q)/(s^2+wn/Q*s+wn^2)
    % iMode=3 used as 2nd-order BPF in SOGI, SOGI_BPF(s)=(wn*s/Q)/(s^2+wn/Q*s+wn^2)
    
    persistent t;
    
    if isempty(t)
        t = zeros(2,3);
    end
    
    wn = 2*pi*fn;
    wc = wn/fQ;

    fT1 = wc*wn*fTs*fTs; 
    fT2 = 2*wc*fTs;
    fT3 = (wn*fTs)^2;
    
    fb1 = fT3+fT2+4;
    fb2 = 2*fT3-8;
    fb3 = fT3-fT2+4;
    
    if (iMode ==1)
        fa1 = fT3;
        fa2 = 2*fT3;
        fa3 = fT3;
    elseif (iMode ==2)
        fa1 = fT1;
        fa2 = 2*fT1;
        fa3 = fT1;
    else
        fa1 = fT2;
        fa2 = 0;
        fa3 = -fT2;
    end
        
%    if(Trigs > 0)
        t(1,1) = u;        
        t(2,1) = (fa1*t(1,1)+fa2*t(1,2)+fa3*t(1,3)-fb2*t(2,2)-fb3*t(2,3))/fb1;
    
        t(1,3) = t(1,2);
        t(1,2) = t(1,1);
        
        t(2,3) = t(2,2);
        t(2,2) = t(2,1);
%     else
%         t(1,1) = t(1,1);        
%         t(2,1) = t(2,1);
%     
%         t(1,3) = t(1,3);
%         t(1,2) = t(1,2);
%         
%         t(2,3) = t(2,3);
%         t(2,2) = t(2,2);
%     end
    
    y = t(2,1);    
end

== matlab function CSI_0313_SDC/AIP1/Subsystem7/Pos Compensation/VIriz_To_PQ_Calc SI Units ==
  data: Vriz input; P output; Q output; Iriz input
function [P, Q] = VIriz_To_PQ(Vriz, Iriz)
    % Vriz and Iriz to calculate the active & reactive power
    % Vriz: Voltage in Re-Im axis
    % Iriz: Current in Re-Im axis
    
    P = 1.5*(Vriz(1)*Iriz(1) + Vriz(2)*Iriz(2))/1000;
    Q = 1.5*(Vriz(2)*Iriz(1) - Vriz(1)*Iriz(2))/1000;
end

== matlab function CSI_0313_SDC/AIP1/Subsystem7/Pos Compensation/VIriz_To_PQ_Calc SI Units1 ==
  data: Vriz input; P output; Q output; Iriz input
function [P, Q] = VIriz_To_PQ(Vriz, Iriz)
    % Vriz and Iriz to calculate the active & reactive power
    % Vriz: Voltage in Re-Im axis
    % Iriz: Current in Re-Im axis
    
    P = 1.5*(Vriz(1)*Iriz(1) + Vriz(2)*Iriz(2))/1000;
    Q = 1.5*(Vriz(2)*Iriz(1) - Vriz(1)*Iriz(2))/1000;
end

== matlab function CSI_0313_SDC/AIP1/Subsystem7/Pos Compensation/RIZ_To_DQ0 ==
  data: RIZ input; DQ0 output; wt input; iAxis parameter
function DQ0 = RIZ_To_DQ0(RIZ,wt,iAxis)
    % Park Transfer from Re-Im axis to DQ0 axis
    DQ0 = [0;0;0];
    if (iAxis == 1)
        DQ0(1) = RIZ(1)*cos(wt)+RIZ(2)*sin(wt);
        DQ0(2) = -RIZ(1)*sin(wt)+RIZ(2)*cos(wt);
    else
        DQ0(1) = RIZ(1)*sin(wt)-RIZ(2)*cos(wt);
        DQ0(2) = RIZ(1)*cos(wt)+RIZ(2)*sin(wt);
    end
end

== matlab function CSI_0313_SDC/AIP1/Subsystem7/Neg seq compensation/RIZ_To_DQ0 ==
  data: RIZ input; DQ0 output; wt input; iAxis parameter
function DQ0 = RIZ_To_DQ0(RIZ,wt,iAxis)
    % Park Transfer from Re-Im axis to DQ0 axis
    DQ0 = [0;0;0];
    if (iAxis == 1)
        DQ0(1) = RIZ(1)*cos(wt)+RIZ(2)*sin(wt);
        DQ0(2) = -RIZ(1)*sin(wt)+RIZ(2)*cos(wt);
    else
        DQ0(1) = RIZ(1)*sin(wt)-RIZ(2)*cos(wt);
        DQ0(2) = RIZ(1)*cos(wt)+RIZ(2)*sin(wt);
    end
end

== matlab function CSI_0313_SDC/AIP1/Subsystem7/Neg seq compensation/RIZ_To_DQ1 ==
  data: RIZ input; DQ0 output; wt input; iAxis parameter
function DQ0 = RIZ_To_DQ0(RIZ,wt,iAxis)
    % Park Transfer from Re-Im axis to DQ0 axis
    DQ0 = [0;0;0];
    if (iAxis == 1)
        DQ0(1) = RIZ(1)*cos(wt)+RIZ(2)*sin(wt);
        DQ0(2) = -RIZ(1)*sin(wt)+RIZ(2)*cos(wt);
    else
        DQ0(1) = RIZ(1)*sin(wt)-RIZ(2)*cos(wt);
        DQ0(2) = RIZ(1)*cos(wt)+RIZ(2)*sin(wt);
    end
end

== matlab function CSI_0313_SDC/AIP1/Subsystem7/PLL/PI Ctrl ==
  data: err input; y output; fKI parameter; fMinLmt parameter; fTs parameter; fMaxLmt parameter; fKP parameter
function y = PICtrl(err, fKI, fMinLmt, fTs, fMaxLmt, fKP)
    % y[n] = y[n-1] + KP*(x[n]-x[n-1]) + (KP*KI*TS*0.5)*(x[n]+x[n-1])
    % err:  error input
    % fKP:   Proportional gain
    % fKI:   Integral Coefficient
    % fMinLmt: Minimum limitation
    % fMaxLmt: Maximum limitation
    % fTs:  Sampling time
    
    % t(1,2) stores x[n],x[n-1]; t(2,2) stores y[n],y[n-1]
    persistent t;      
    if isempty(t)           % Initialization
        t = zeros(2,2);
    end

%     if(Trig > 0)
        t(1,1) = err;
        t(2,1) = t(2,2) + fKP*(t(1,1)-t(1,2)) + fKP*fKI*0.5*(t(1,1)+t(1,2))*fTs;   
    
        if (t(2,1) < fMinLmt)
            t(2,1) = fMinLmt;
        elseif (t(2,1) > fMaxLmt)
            t(2,1) = fMaxLmt;
        end
        t(1,2) = t(1,1);
        t(2,2) = t(2,1);
%     else
%         t(1,1) = t(1,1);
%         t(2,1) = t(2,1);   
%         t(1,2) = t(1,2);
%         t(2,2) = t(2,2);
%     end
    
    y = t(2,1);
end

== matlab function CSI_0313_SDC/AIP1/Subsystem7/PLL/Integral ==
  data: u input; fGain parameter; fTs parameter; y output
function y  = Integral(u, fGain, fTs)
    % y[n] = y[n-1] + (TS*0.5)*(x[n]+x[n-1])
    % u:     input
    % fGain: Gain
    % fTs:  Sampling time
    
    % t(1,2) stores x[n],x[n-1]; t(2,2) stores y[n],y[n-1]
    persistent t;      
    if isempty(t)           % Initialization
        t = zeros(2,2);
    end
%     if(Trig > 0)
        t(1,1) = u;
        t(2,1) = t(2,2) + fGain*0.5*fTs*(t(1,1)+t(1,2));   

        t(1,2) = t(1,1);
        t(2,2) = t(2,1);
%     else
%         t(1,1) = t(1,1);
%         t(2,1) = t(2,1);   
% 
%         t(1,2) = t(1,2);
%         t(2,2) = t(2,2);
%     end
    y = t(2,1);
end

== matlab function CSI_0313_SDC/AIP1/Subsystem7/Neg seq compensation/PI Ctrl1 ==
  data: err input; y output; fKI parameter; fMinLmt parameter; fTs parameter; fMaxLmt parameter; fKP parameter
function y = PICtrl(err, fKI, fMinLmt, fTs, fMaxLmt, fKP)
    % y[n] = y[n-1] + KP*(x[n]-x[n-1]) + (KP*KI*TS*0.5)*(x[n]+x[n-1])
    % err:  error input
    % fKP:   Proportional gain
    % fKI:   Integral Coefficient
    % fMinLmt: Minimum limitation
    % fMaxLmt: Maximum limitation
    % fTs:  Sampling time
    
    % t(1,2) stores x[n],x[n-1]; t(2,2) stores y[n],y[n-1]
    persistent t;      
    if isempty(t)           % Initialization
        t = zeros(2,2);
    end
    
%     if(Trig > 0)
        t(1,1) = err;
        t(2,1) = t(2,2) + fKP*(t(1,1)-t(1,2)) + fKP*fKI*0.5*(t(1,1)+t(1,2))*fTs;   
    
        if (t(2,1) < fMinLmt)
            t(2,1) = fMinLmt;
        elseif (t(2,1) > fMaxLmt)
            t(2,1) = fMaxLmt;
        end
    
        t(1,2) = t(1,1);
        t(2,2) = t(2,1);
%     else
%         t(1,1) = t(1,1);
%         t(2,1) = t(2,1);      
%         t(1,2) = t(1,2);
%         t(2,2) = t(2,2);
%     end
    y = t(2,1);
end

== matlab function CSI_0313_SDC/AIP1/Subsystem7/Neg seq compensation/PI Ctrl2 ==
  data: err input; y output; fKI parameter; fMinLmt parameter; fTs parameter; fMaxLmt parameter; fKP parameter
function y = PICtrl(err, fKI, fMinLmt, fTs, fMaxLmt, fKP)
    % y[n] = y[n-1] + KP*(x[n]-x[n-1]) + (KP*KI*TS*0.5)*(x[n]+x[n-1])
    % err:  error input
    % fKP:   Proportional gain
    % fKI:   Integral Coefficient
    % fMinLmt: Minimum limitation
    % fMaxLmt: Maximum limitation
    % fTs:  Sampling time
    
    % t(1,2) stores x[n],x[n-1]; t(2,2) stores y[n],y[n-1]
    persistent t;      
    if isempty(t)           % Initialization
        t = zeros(2,2);
    end
    
%     if(Trig > 0)
        t(1,1) = err;
        t(2,1) = t(2,2) + fKP*(t(1,1)-t(1,2)) + fKP*fKI*0.5*(t(1,1)+t(1,2))*fTs;   
    
        if (t(2,1) < fMinLmt)
            t(2,1) = fMinLmt;
        elseif (t(2,1) > fMaxLmt)
            t(2,1) = fMaxLmt;
        end
    
        t(1,2) = t(1,1);
        t(2,2) = t(2,1);
%     else
%         t(1,1) = t(1,1);
%         t(2,1) = t(2,1);      
%         t(1,2) = t(1,2);
%         t(2,2) = t(2,2);
%     end
    y = t(2,1);
end

== matlab function CSI_0313_SDC/AIP1/Subsystem7/Zero seq compensation/PR Ctrl1 ==
  data: err input; y output; ffc input; fP parameter; fQ parameter; fTs parameter
function y = PRCtrl(err, ffc, fP, fQ, fTs)
    % PR regulation with variant frequency input
    % y[n] = (fa1*x[n]+fa2*x[n-1]+fa3*x[n-2]-fb2*y[n-1]-fb3*y[n-2])/fb1
    % err:  error input
    % ffc:  Natural frequency
    % fP:   Proportional gain
    % fQ:   Quality factor
    % fTs:  Sampling time
    
    % t(1,3) stores x[n],x[n-1],x[n-2]; t(2,3) stores y[n],y[n-1],y[n-2]
    persistent t;      
    if isempty(t)           % Initialization
        t = zeros(2,3);
    end

    fwc = 2*pi*ffc;
    fw0 = fwc/fQ;
    
    fT1 = 2*fw0*fTs;            
    fT2 = (fwc*fTs)^2;  

    fa1 = (4+fT1+fT2)*fP;
    fa2 = (2*fT2-8)*fP;
    fa3 = (4-fT1+fT2)*fP;
    fb1 = 4+fT2;
    fb2 = 2*fT2-8;
    fb3 = 4+fT2;
%     if(Trig > 0)
        t(1,1) = err;
        t(2,1) = (fa1*t(1,1)+fa2*t(1,2)+fa3*t(1,3)-fb2*t(2,2)-fb3*t(2,3))/fb1;     
        
        t(1,3) = t(1,2);
        t(1,2) = t(1,1);
 
        t(2,3) = t(2,2);
        t(2,2) = t(2,1);
%     else
%         t(1,1) = t(1,1);
%         t(2,1) = t(2,1);     
%         
%         t(1,3) = t(1,3);
%         t(1,2) = t(1,2);
%  
%         t(2,3) = t(2,3);
%         t(2,2) = t(2,2);
%         
%     end
    y = t(2,1);
end

== matlab function CSI_0313_SDC/AIP1/Subsystem7/Pos Compensation1/PI Ctrl1 ==
  data: err input; y output; fKI parameter; fMinLmt parameter; fTs parameter; fMaxLmt parameter; fKP parameter
function y = PICtrl(err, fKI, fMinLmt, fTs, fMaxLmt, fKP)
    % y[n] = y[n-1] + KP*(x[n]-x[n-1]) + (KP*KI*TS*0.5)*(x[n]+x[n-1])
    % err:  error input
    % fKP:   Proportional gain
    % fKI:   Integral Coefficient
    % fMinLmt: Minimum limitation
    % fMaxLmt: Maximum limitation
    % fTs:  Sampling time
    
    % t(1,2) stores x[n],x[n-1]; t(2,2) stores y[n],y[n-1]
    persistent t;      
    if isempty(t)           % Initialization
        t = zeros(2,2);
    end
    
%     if(Trig > 0)
        t(1,1) = err;
        t(2,1) = t(2,2) + fKP*(t(1,1)-t(1,2)) + fKP*fKI*0.5*(t(1,1)+t(1,2))*fTs;   
    
        if (t(2,1) < fMinLmt)
            t(2,1) = fMinLmt;
        elseif (t(2,1) > fMaxLmt)
            t(2,1) = fMaxLmt;
        end
    
        t(1,2) = t(1,1);
        t(2,2) = t(2,1);
%     else
%         t(1,1) = t(1,1);
%         t(2,1) = t(2,1);      
%         t(1,2) = t(1,2);
%         t(2,2) = t(2,2);
%     end
    y = t(2,1);
end

== matlab function CSI_0313_SDC/AIP1/Subsystem7/Neg seq compensation/DQ0_To_RIZ ==
  data: DQ0 input; RIZ output; wt input; iAxis parameter
function RIZ = DQ0_To_RIZ(DQ0,wt,iAxis)
    % Inverse Park Transfer from DQ0 axis to Re-Im axis
    RIZ = [0;0;0];
    if (iAxis == 1)
        RIZ(1) = DQ0(1)*cos(wt)-DQ0(2)*sin(wt);
        RIZ(2) = DQ0(1)*sin(wt)+DQ0(2)*cos(wt);
    else
        RIZ(1) = DQ0(1)*sin(wt)+DQ0(2)*cos(wt);
        RIZ(2) = -DQ0(1)*cos(wt)+DQ0(2)*sin(wt);
    end
end

== matlab function CSI_0313_SDC/AIP1/Subsystem7/Pos Compensation/PQ_Vriz_To_Iriz pu Standard ==
  data: P input; Q input; Vriz input size=3; Iriz output size=3; Ibase parameter; wt input
function Iriz = PQ_V_To_Iriz(P, Q, Vriz,Ibase,wt)
    % PQ and Vriz to calculate the Iriz
    % Vriz: Voltage in Re-Im axis
    % Iriz: Current in Re-Im axis
    % The Vamp calculation without coefficient 1.5
    Iriz = [0;0;0];
    Vamp_squr = Vriz(1)*Vriz(1) + Vriz(2)*Vriz(2);
    if (Vamp_squr <= 0)
        Vamp_squr = 1;
    end
    Iriz(1) = 2000/3*(Vriz(1)*P + Vriz(2)*Q)/Vamp_squr;
    Iriz(2) = 2000/3*(Vriz(2)*P - Vriz(1)*Q)/Vamp_squr;
    
    Id = Iriz(1)*sin(wt)-Iriz(2)*cos(wt);
    Iq = Iriz(1)*cos(wt)+Iriz(2)*sin(wt);
%     Iamp = sqrt(Id*Id+Iq*Iq);
%     Id = Id/Iamp*Ibase;
%     Iq = Iq/Iamp*Ibase;
    if (Id >= Ibase)
        Id = Ibase;
    elseif (Id <= -Ibase)
        Id = -Ibase;
    end
    if (Iq >= Ibase)
        Iq = Ibase;
    elseif (Iq <= -Ibase)
        Iq = -Ibase;
    end
    Iriz(1) = Id *sin(wt)+Iq*cos(wt);
    Iriz(2) = -Id *cos(wt)+Iq*sin(wt);
    Iriz(3) = 0;
end

== matlab function CSI_0313_SDC/AIP1/Subsystem7/Pos Compensation/PI Ctrl2 ==
  data: err input; y output; fKI parameter; fMinLmt parameter; fTs parameter; fMaxLmt parameter; fKP parameter
function y = PICtrl(err, fKI, fMinLmt, fTs, fMaxLmt, fKP)
    % y[n] = y[n-1] + KP*(x[n]-x[n-1]) + (KP*KI*TS*0.5)*(x[n]+x[n-1])
    % err:  error input
    % fKP:   Proportional gain
    % fKI:   Integral Coefficient
    % fMinLmt: Minimum limitation
    % fMaxLmt: Maximum limitation
    % fTs:  Sampling time
    
    % t(1,2) stores x[n],x[n-1]; t(2,2) stores y[n],y[n-1]
    persistent t;      
    if isempty(t)           % Initialization
        t = zeros(2,2);
    end
    
%     if(Trig > 0)
        t(1,1) = err;
        t(2,1) = t(2,2) + fKP*(t(1,1)-t(1,2)) + fKP*fKI*0.5*(t(1,1)+t(1,2))*fTs;   
    
        if (t(2,1) < fMinLmt)
            t(2,1) = fMinLmt;
        elseif (t(2,1) > fMaxLmt)
            t(2,1) = fMaxLmt;
        end
    
        t(1,2) = t(1,1);
        t(2,2) = t(2,1);
%     else
%         t(1,1) = t(1,1);
%         t(2,1) = t(2,1);      
%         t(1,2) = t(1,2);
%         t(2,2) = t(2,2);
%     end
    y = t(2,1);
end

== matlab function CSI_0313_SDC/AIP1/Subsystem7/Pos Compensation/PI Ctrl1 ==
  data: err input; y output; fKI parameter; fMinLmt parameter; fTs parameter; fMaxLmt parameter; fKP parameter
function y = PICtrl(err, fKI, fMinLmt, fTs, fMaxLmt, fKP)
    % y[n] = y[n-1] + KP*(x[n]-x[n-1]) + (KP*KI*TS*0.5)*(x[n]+x[n-1])
    % err:  error input
    % fKP:   Proportional gain
    % fKI:   Integral Coefficient
    % fMinLmt: Minimum limitation
    % fMaxLmt: Maximum limitation
    % fTs:  Sampling time
    
    % t(1,2) stores x[n],x[n-1]; t(2,2) stores y[n],y[n-1]
    persistent t;      
    if isempty(t)           % Initialization
        t = zeros(2,2);
    end
    
%     if(Trig > 0)
        t(1,1) = err;
        t(2,1) = t(2,2) + fKP*(t(1,1)-t(1,2)) + fKP*fKI*0.5*(t(1,1)+t(1,2))*fTs;   
    
        if (t(2,1) < fMinLmt)
            t(2,1) = fMinLmt;
        elseif (t(2,1) > fMaxLmt)
            t(2,1) = fMaxLmt;
        end
    
        t(1,2) = t(1,1);
        t(2,2) = t(2,1);
%     else
%         t(1,1) = t(1,1);
%         t(2,1) = t(2,1);      
%         t(1,2) = t(1,2);
%         t(2,2) = t(2,2);
%     end
    y = t(2,1);
end

== matlab function CSI_0313_SDC/AIP1/Subsystem5/PLL/ABC_To_RIZ ==
  data: ABC input size=3; RIZ output size=3
function RIZ = ABC_To_RIZ(ABC)
    % Clarke Transfer from ABC axis to Re-Im axis
    RIZ = [0;0;0];
    RIZ(1) = (2*ABC(1)-ABC(2)-ABC(3))/3;
    RIZ(2) = sqrt(3)*(ABC(2)-ABC(3))/3;
    RIZ(3) = (ABC(1)+ABC(2)+ABC(3))/3;
end

== matlab function CSI_0313_SDC/AIP1/Subsystem5/PLL/Integral ==
  data: u input; fGain parameter; fTs parameter; y output
function y  = Integral(u, fGain, fTs)
    % y[n] = y[n-1] + (TS*0.5)*(x[n]+x[n-1])
    % u:     input
    % fGain: Gain
    % fTs:  Sampling time
    
    % t(1,2) stores x[n],x[n-1]; t(2,2) stores y[n],y[n-1]
    persistent t;      
    if isempty(t)           % Initialization
        t = zeros(2,2);
    end
%     if(Trig > 0)
        t(1,1) = u;
        t(2,1) = t(2,2) + fGain*0.5*fTs*(t(1,1)+t(1,2));   

        t(1,2) = t(1,1);
        t(2,2) = t(2,1);
%     else
%         t(1,1) = t(1,1);
%         t(2,1) = t(2,1);   
% 
%         t(1,2) = t(1,2);
%         t(2,2) = t(2,2);
%     end
    y = t(2,1);
end
